simulink model "untitled2"  (R2023b)
settings: Solver=VariableStepAuto  StartTime=0.0  StopTime=10.0  RelTol=1e-3
settings Model: Creator=a2  LastModifiedBy=a2

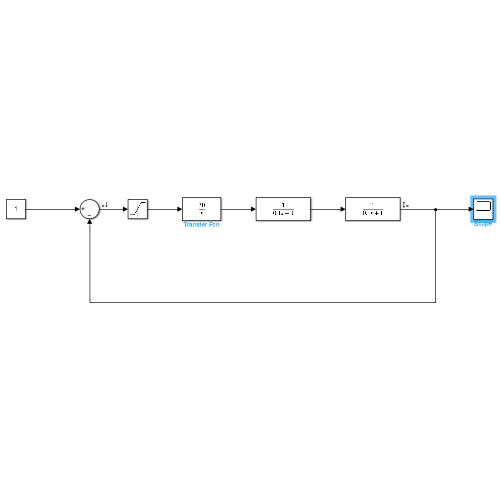
[thumbnail: Simulink's stored preview of the top-level diagram]
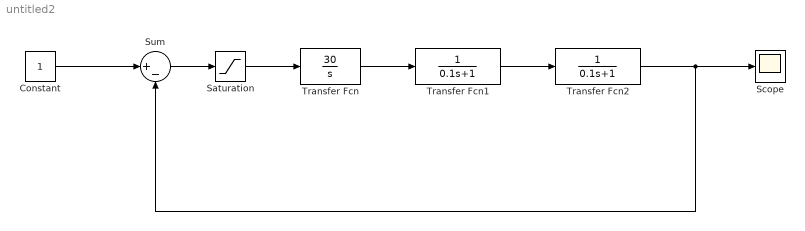
== system untitled2 ==
  Constant : Constant
  Saturation : Saturate  UpperLimit=10  LowerLimit=-10
  Scope : Scope
  Sum : Sum  Inputs=|+-
  Transfer Fcn : TransferFcn  Numerator=[30]  Denominator=[1 0]
  Transfer Fcn1 : TransferFcn  Denominator=[0.1 1]
  Transfer Fcn2 : TransferFcn  Denominator=[0.1 1]
  wires:
  Constant/1 -> Sum/1
  Sum/1 -> Saturation/1
  Transfer Fcn/1 -> Transfer Fcn1/1
  Transfer Fcn1/1 -> Transfer Fcn2/1
  Transfer Fcn2/1 -> Sum/2, Scope/1
  Saturation/1 -> Transfer Fcn/1
